simulink model "untitled"  (R2016a)
settings: Solver=VariableStepAuto  StartTime=0.0  StopTime=20.0  RelTol=1e-3
settings Model: Creator=Student  LastModifiedBy=Student

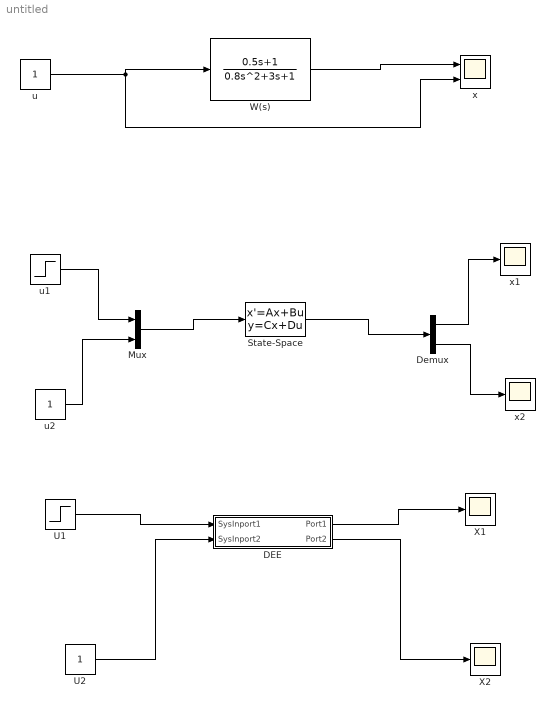
== system untitled ==
  DEE : Subsystem  mask(Differential Equation Editor (DEE)){}
      settings: OpenFcn=diffeqed
      mask Display: disp('Differential Equation\n Editor')
  Demux : Demux  Outputs=2
  Mux : Mux  Inputs=2
  State-Space : StateSpace  A=[-1 -1;1 0]  B=[1 0;0 1]  C=[1 0;0 1]  D=[0 0;0 0]  X0=[0 0]
  U1 : Step  SampleTime=0
  U2 : Constant
  W(s) : TransferFcn  Numerator=[0.5 1]  Denominator=[0.8 3 1]
  X1 : Scope
  X2 : Scope
  u : Constant
  u1 : Step  SampleTime=0
  u2 : Constant
  x : Scope  NumInputPorts=2
  x1 : Scope
  x2 : Scope
  wires:
  u/1 -> x/2, W(s)/1
  W(s)/1 -> x/1
  u1/1 -> Mux/1
  u2/1 -> Mux/2
  Mux/1 -> State-Space/1
  State-Space/1 -> Demux/1
  Demux/1 -> x1/1
  Demux/2 -> x2/1
  U1/1 -> DEE/1(SysInport1)
  U2/1 -> DEE/2(SysInport2)
  DEE/1(Port1) -> X1/1
  DEE/2(Port2) -> X2/1

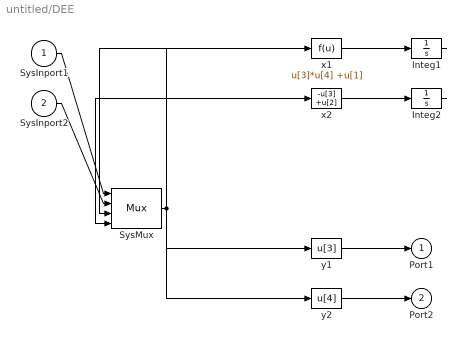
== system untitled/DEE ==
  SysInport1 : Inport
  SysInport2 : Inport  Port=2
  Integ1 : Integrator
  Integ2 : Integrator
  SysMux : Mux
  x1 : Fcn  Expr=u[3]*u[4] +u[1]
  x2 : Fcn  Expr=-u[3] +u[2]
  y1 : Fcn  Expr=u[3]
  y2 : Fcn  Expr=u[4]
  Port1 : Outport
  Port2 : Outport  Port=2
  wires:
  SysInport1/1 -> SysMux/1
  SysInport2/1 -> SysMux/2
  SysMux/1 -> x1/1, x2/1, y1/1, y2/1
  x1/1 -> Integ1/1
  Integ1/1 -> SysMux/3
  x2/1 -> Integ2/1
  Integ2/1 -> SysMux/4
  y1/1 -> Port1/1
  y2/1 -> Port2/1
